simulink model "Stoergroessensprung"  (R2021b)
settings: Solver=ode1  StartTime=0.0  StopTime=700  FixedStep=0.001  RelTol=1e-3
values from neighbouring files (symbols this model uses):
  KdKom = 0    [Ausarbeitung.m]
  KdLa = TdLa*KrLa    [Ausarbeitung.m]
  KdStr = 0    [Ausarbeitung.m]
  KdTsum = TdTsum*KrTsum    [Ausarbeitung.m]
  KiKom = sys(500)-sys(1)    [Ausarbeitung.m]
  KiLa = KrLa/TiLa    [Ausarbeitung.m]
  KiStr = KrStr/TiStr    [Ausarbeitung.m]
  KiTsum = KrTsum/TiTsum    [Ausarbeitung.m]
  KrKom = sys(1)    [Ausarbeitung.m]
  KrLa = 1/KpY    [Ausarbeitung.m]
  KrStr = 1/KpY + (k^2+1)/2*k    [Ausarbeitung.m]
  KrTsum = 1/KpY    [Ausarbeitung.m]
libraries: slpidlib x8
settings Model: Creator=Basti  LastModifiedBy=the_main_notebook

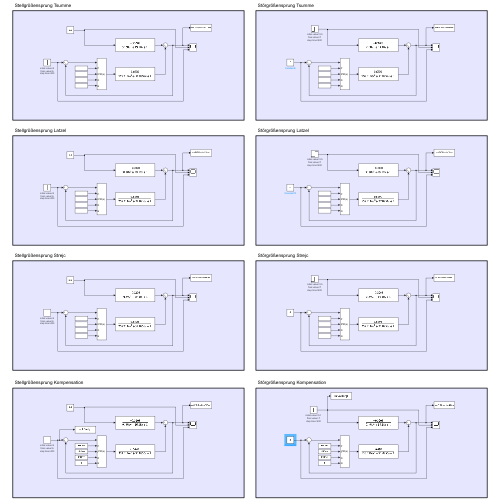
[thumbnail: Simulink's stored preview of the top-level diagram]
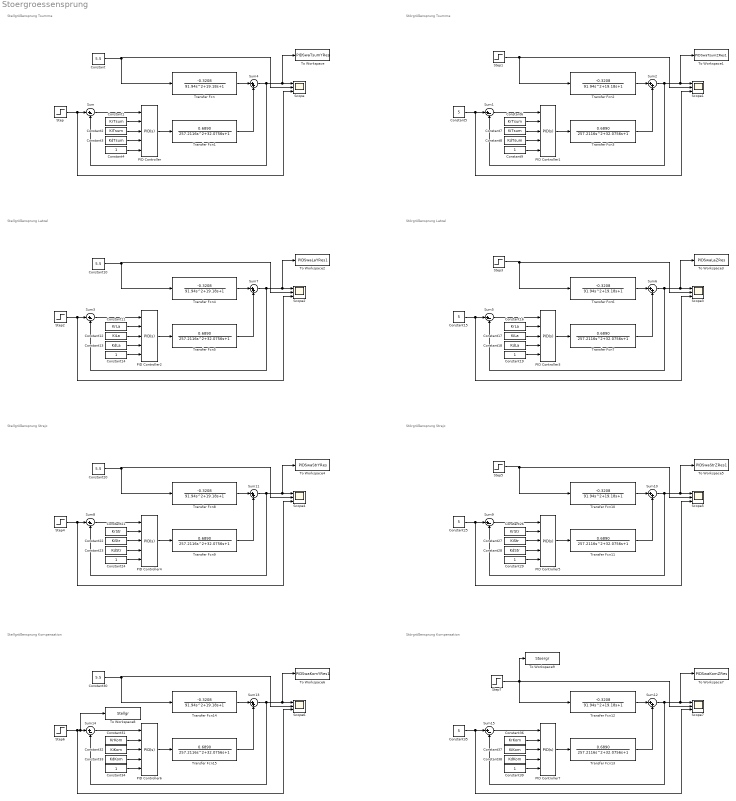
== system Stoergroessensprung ==
  note: Stellgrößensprung Tsumme
  note: Störgrößensprung Tsumme
  note: Störgrößensprung Latzel
  note: Stellgrößensprung Latzel
  note: Stellgrößensprung Strejc
  note: Störgrößensprung Strejc
  note: Störgrößensprung Kompensation
  note: Stellgrößensprung Kompensation
  Constant{,10,20,30} (4 alike) : Constant  Value=5.5
  Constant1 : Constant  Value=KrTsum
  Constant11 : Constant  Value=KrLa
  Constant12 : Constant  Value=KiLa
  Constant13 : Constant  Value=KdLa
  Constant{4,9,14,19,24,29,34,39} (8 alike) : Constant
  Constant{5,15,25,35} (4 alike) : Constant  Value=5
  Constant16 : Constant  Value=KrLa
  Constant17 : Constant  Value=KiLa
  Constant18 : Constant  Value=KdLa
  Constant2 : Constant  Value=KiTsum
  Constant21 : Constant  Value=KrStr
  Constant22 : Constant  Value=KiStr
  Constant23 : Constant  Value=KdStr
  Constant26 : Constant  Value=KrStr
  Constant27 : Constant  Value=KiStr
  Constant28 : Constant  Value=KdStr
  Constant3 : Constant  Value=KdTsum
  Constant31 : Constant  Value=KrKom
  Constant32 : Constant  Value=KiKom
  Constant33 : Constant  Value=KdKom
  Constant36 : Constant  Value=KrKom
  Constant37 : Constant  Value=KiKom
  Constant38 : Constant  Value=KdKom
  Constant6 : Constant  Value=KrTsum
  Constant7 : Constant  Value=KiTsum
  Constant8 : Constant  Value=KdTsum
  PID Controller{,1..7} (8 alike) : slpidlib/PID Controller  Controller=PID  Form=Parallel  TimeDomain=Continuous-time  UseExternalTs=off  SampleTime=-1  IntegratorMethod=Forward Euler  FilterMethod=Forward Euler  ControllerParametersSource=external  P=1  I=1  D=0  UseFilter=on  N=100  TunerSelectOption=Transfer Function Based (PID Tuner App)  InitialConditionSource=internal  InitialConditionForIntegrator=0  InitialConditionForFilter=0  DifferentiatorICPrevScaledInput=0  ExternalReset=none  TrackingMode=off  Kt=1  LimitOutput=off  SatLimitsSource=internal  UpperSaturationLimit=inf  LowerSaturationLimit=-inf  LinearizeAsGain=on  AntiWindupMode=none  Kb=1  POutMin=[]  POutMax=[]  IOutMin=[]  IOutMax=[]  DOutMin=[]  DOutMax=[]  NOutMin=[]  NOutMax=[]  SumOutMin=[]  SumOutMax=[]  SaturationOutMin=[]  SaturationOutMax=[]  PParamMin=[]  PParamMax=[]  IParamMin=[]  IParamMax=[]  DParamMin=[]  DParamMax=[]  NParamMin=[]  NParamMax=[]  KbParamMin=[]  KbParamMax=[]  KtParamMin=[]  KtParamMax=[]  KbOutMin=[]  KbOutMax=[]  KtOutMin=[]  KtOutMax=[]  IntegratorOutMin=[]  IntegratorOutMax=[]  FilterOutMin=[]  FilterOutMax=[]  SumI1OutMin=[]  SumI1OutMax=[]  SumI2OutMin=[]  SumI2OutMax=[]  SumI3OutMin=[]  SumI3OutMax=[]  SumI4OutMin=[]  SumI4OutMax=[]  SumDOutMin=[]  SumDOutMax=[]  DifferentiatorOutMin=[]  DifferentiatorOutMax=[]  FilterDiffOutCoefMin=[]  FilterDiffOutCoefMax=[]  ReciprocalOutMin=[]  ReciprocalOutMax=[]  SumDenOutMin=[]  SumDenOutMax=[]  SumNumOutMin=[]  SumNumOutMax=[]  DivideOutMin=[]  DivideOutMax=[]  UdiffTsProdOutMin=[]  UdiffTsProdOutMax=[]  NTsProdOutMin=[]  NTsProdOutMax=[]  UintegralTsProdOutMin=[]  UintegralTsProdOutMax=[]  UngainTsProdOutMin=[]  UngainTsProdOutMax=[]  IntegratorContinuousStateAttributes=''  IntegratorStateMustResolveToSignalObject=off  IntegratorRTWStateStorageClass=Auto  FilterContinuousStateAttributes=''  FilterStateMustResolveToSignalObject=off  FilterRTWStateStorageClass=Auto  ParallelPVariant=ExternalParameters  IdealPVariant=Disabled  IVariant=ExternalParameters  DVariant=ExternalParameters  IntegratorVariant=Continuous  SatVariant=Disabled  AWVariant=Passthrough  PCopyVariant=Disabled  TRVariant=Disabled  FdbkBlocksVariant=Forward  IdealPFdbkVariant=Disabled  SatFdbkVariant=Disabled  DerivativeFilterVariant=ContFilter  NVariant=ExternalParameters  NCopyVariant=Disabled  FilterICVariant=InternalICsFilter  IntegratorICVariant=InternalICs  ExternalResetVariant=Disabled  TRSumVariant=Passthrough  SumFdbkVariant=Disabled  SumVariant=Sum_PID  TsampFilterVariant=InternalTs  TsampNgainVariant=Passthrough  TsampIntegralVariant=Passthrough  ExternalSaturationOutDataTypeStr=Inherit: Same as second input
  Scope{,1..7} (8 alike) : Scope  NumInputPorts=3
  Step{,2,4,6} (4 alike) : Step  Time=400  Before=4  After=6  SampleTime=0
      settings: AttributesFormatString=initial value=%<Before>\nfinal value=%<After>\nstep time=%<Time>
  Step{1,3,5,7} (4 alike) : Step  Time=400  Before=5.5  After=7  SampleTime=0
      settings: AttributesFormatString=initial value=%<Before>\nfinal value=%<After>\nstep time=%<Time>
  Sum{,1,3,5,8..9,14..15} (8 alike) : Sum  Inputs=|+-
  Sum{2,4,6..7,10..13} (8 alike) : Sum  Inputs=|++
  To Workspace : ToWorkspace  VariableName=PIDSwaTsumYRes  SampleTime=-1
  To Workspace1 : ToWorkspace  VariableName=PIDSwaTsumZRes1  SampleTime=-1
  To Workspace2 : ToWorkspace  VariableName=PIDSwaLaYRes1  SampleTime=-1
  To Workspace3 : ToWorkspace  VariableName=PIDSwaLaZRes  SampleTime=-1
  To Workspace4 : ToWorkspace  VariableName=PIDSwaStrYRes  SampleTime=-1
  To Workspace5 : ToWorkspace  VariableName=PIDSwaStrZRes1  SampleTime=-1
  To Workspace6 : ToWorkspace  VariableName=PIDSwaKomYRes1  SampleTime=-1
  To Workspace7 : ToWorkspace  VariableName=PIDSwaKomZRes  SampleTime=-1
  To Workspace8 : ToWorkspace  VariableName=Stellgr  SampleTime=-1
  To Workspace9 : ToWorkspace  VariableName=Stoergr  SampleTime=-1
  Transfer Fcn{,2,4,6,8,10,12,14} (8 alike) : TransferFcn  Numerator=[-0.3208]  Denominator=[91.94 19.18 1]
  Transfer Fcn{1,3,5,7,9,11,13,15} (8 alike) : TransferFcn  Numerator=[0.6890]  Denominator=[257.2116 32.0756 1]
  wires:
  Step/1 -> Scope/3, Sum/1
  PID Controller/1 -> Transfer Fcn1/1
  Transfer Fcn/1 -> Sum4/1
  Transfer Fcn1/1 -> Sum4/2
  Constant/1 -> Scope/2, Transfer Fcn/1
  Sum4/1 -> Sum/2, To Workspace/1, Scope/1
  Sum/1 -> PID Controller/1
  Constant1/1 -> PID Controller/2
  Constant3/1 -> PID Controller/4
  Constant2/1 -> PID Controller/3
  Constant4/1 -> PID Controller/5
  Constant9/1 -> PID Controller1/5
  Constant7/1 -> PID Controller1/3
  Constant8/1 -> PID Controller1/4
  PID Controller1/1 -> Transfer Fcn3/1
  Constant6/1 -> PID Controller1/2
  Transfer Fcn2/1 -> Sum2/1
  Step1/1 -> Transfer Fcn2/1, Scope1/2
  Sum2/1 -> Sum1/2, To Workspace1/1, Scope1/1
  Sum1/1 -> PID Controller1/1
  Transfer Fcn3/1 -> Sum2/2
  Constant5/1 -> Scope1/3, Sum1/1
  Sum6/1 -> Sum5/2, To Workspace3/1, Scope3/1
  Constant15/1 -> Scope3/3, Sum5/1
  Transfer Fcn7/1 -> Sum6/2
  Sum5/1 -> PID Controller3/1
  Constant16/1 -> PID Controller3/2
  Constant19/1 -> PID Controller3/5
  Constant18/1 -> PID Controller3/4
  Constant17/1 -> PID Controller3/3
  Transfer Fcn6/1 -> Sum6/1
  Constant10/1 -> Scope2/2, Transfer Fcn4/1
  Step3/1 -> Transfer Fcn6/1, Scope3/2
  Constant14/1 -> PID Controller2/5
  Step2/1 -> Scope2/3, Sum3/1
  Constant12/1 -> PID Controller2/3
  Constant13/1 -> PID Controller2/4
  PID Controller2/1 -> Transfer Fcn5/1
  Constant11/1 -> PID Controller2/2
  Transfer Fcn4/1 -> Sum7/1
  Sum7/1 -> Sum3/2, To Workspace2/1, Scope2/1
  PID Controller3/1 -> Transfer Fcn7/1
  Sum3/1 -> PID Controller2/1
  Transfer Fcn5/1 -> Sum7/2
  Transfer Fcn8/1 -> Sum11/1
  Sum8/1 -> PID Controller4/1
  PID Controller4/1 -> Transfer Fcn9/1
  Step4/1 -> Scope4/3, Sum8/1
  Sum11/1 -> Sum8/2, To Workspace4/1, Scope4/1
  Constant22/1 -> PID Controller4/3
  Constant24/1 -> PID Controller4/5
  Constant20/1 -> Scope4/2, Transfer Fcn8/1
  Constant21/1 -> PID Controller4/2
  Sum9/1 -> PID Controller5/1
  Step5/1 -> Transfer Fcn10/1, Scope5/2
  Transfer Fcn10/1 -> Sum10/1
  Constant29/1 -> PID Controller5/5
  Transfer Fcn9/1 -> Sum11/2
  Transfer Fcn11/1 -> Sum10/2
  Sum10/1 -> Sum9/2, To Workspace5/1, Scope5/1
  Constant23/1 -> PID Controller4/4
  Constant25/1 -> Scope5/3, Sum9/1
  Constant26/1 -> PID Controller5/2
  Constant27/1 -> PID Controller5/3
  PID Controller5/1 -> Transfer Fcn11/1
  Constant28/1 -> PID Controller5/4
  Constant35/1 -> Scope7/3, Sum15/1
  Constant38/1 -> PID Controller7/4
  Constant33/1 -> PID Controller6/4
  Constant37/1 -> PID Controller7/3
  Constant36/1 -> PID Controller7/2
  PID Controller7/1 -> Transfer Fcn13/1
  Transfer Fcn12/1 -> Sum12/1
  Transfer Fcn15/1 -> Sum13/2
  Sum12/1 -> Sum15/2, To Workspace7/1, Scope7/1
  Transfer Fcn13/1 -> Sum12/2
  Constant39/1 -> PID Controller7/5
  Sum15/1 -> PID Controller7/1
  Step7/1 -> To Workspace9/1, Scope7/2, Transfer Fcn12/1
  Constant31/1 -> PID Controller6/2
  Constant30/1 -> Scope6/2, Transfer Fcn14/1
  Constant32/1 -> PID Controller6/3
  Sum13/1 -> Sum14/2, To Workspace6/1, Scope6/1
  Constant34/1 -> PID Controller6/5
  Step6/1 -> Scope6/3, To Workspace8/1, Sum14/1
  Sum14/1 -> PID Controller6/1
  PID Controller6/1 -> Transfer Fcn15/1
  Transfer Fcn14/1 -> Sum13/1
